simulink model "autoTakeoff"  (R2015a)
settings: Solver=ode45  StartTime=0.0  StopTime=inf  FixedStep=0.01  RelTol=1e-3
libraries: simulink x8, dspindex x8, dspnetwork x3, aerolibconvert2 x1, IMU_Library x1, GPS_Library x1, realtime_pacer_lib x1, etargetslib x1
settings Model: xpc_rtwmakecfg_data=_xpcnblib__xpcetherlib__xpcether8255xlib__xpcetherGbElib__xpciplib_  ParamWorkspaceSource=ReferencedWorkspace  CovSFcnEnable=off  Creator=abdkadma  LastModifiedBy=theth
settings OptimizationCC: InlineParams=on  InlineInvariantSignals=on  EnhancedBackFolding=on  ExpressionDepthLimit=2147483647  EfficientFloat2IntCast=on  SimCompilerOptimization=on
settings DebuggingCC: UnderspecifiedInitializationDetection=Classic  MergeDetectMultiDrivingBlocksExec=none  SolverPrmCheckMsg=warning  StateNameClashWarn=warning
settings RTWCC: RTWCompilerOptimization=on  CheckMdlBeforeBuild=Warning
settings GRTTargetCC: MatFileLogging=off  SupportNonFinite=off

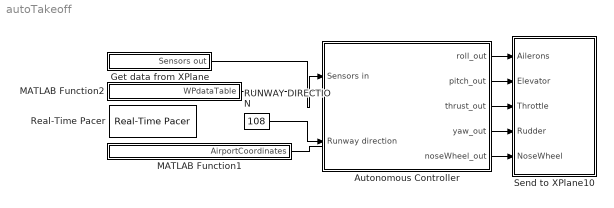
== system autoTakeoff ==
  "Autonomous Controller " : Subsystem
  Get data from XPlane : Subsystem  Description=|  TreatAsAtomicUnit=on  mask(Get Data from Xplane10){remoteURL='127.0.0.1', localPort=49005, sampletime=0.02}
      | Done by: Mohamed Abdelkader
      | Contact for updates: mohamedashraf123@gmail.com
      mask prompts: remoteURL "Remote IP address ('0.0.0.0' to accept all):(default='127.0.0.1')"; localPort "Local IP port: that Xplane10 sends to (default=49005)"; sampletime "Sampling time (seconds), how frequenlty to capture data from Xplane. Don't set to low as it might not be able to capture the smaples from Xplane. Default is 0.02 assuming the UDP rate in Xplane is set to 50 sample per second"
      mask help:
      | Get Data from X-Plane10
      | * make sure you configure the right port
      | and the right IP address
      mask TypeOptions remoteURL: UDP Receive1/remoteURL
      mask TypeOptions localPort: UDP Receive1/localPort
      mask TypeOptions sampletime: UDP Receive1/sampletime
  MATLAB Function1 : MATLAB Function  TreatAsAtomicUnit=on
  MATLAB Function2 : MATLAB Function  TreatAsAtomicUnit=on
  RUNWAY DIRECTION : Constant  Value=108
  Real-Time Pacer : realtime_pacer_lib/Real-Time Pacer  simTimePerRealTime=1
  Send to XPlane10 : Subsystem  Description=|  mask(Send Commands to X-Plane 10){remoteURL='127.0.0.1', remotePort=49000}
      | Done by: Mohamed Abdelkader
      | Contact for updates: mohamedashraf123@gmail.com
      mask prompts: remoteURL "Remote IP address (default='127.0.0.1'): X-Plane10 IP"; remotePort "Remote IP port:X-Plane10 port(default=49000)"
      mask help:
      | Sends Control Surfaces Commands to Xplane10
      | Throttle in [0,1]
      | Elevator, Ailerons, rudder, nosewheel in [-1,1]
      mask TypeOptions remoteURL: UDP Send/remoteURL
      mask TypeOptions remotePort: UDP Send/remotePort
  wires:
  "Autonomous Controller "/1(roll_out) -> Send to XPlane10/1(Ailerons)
  "Autonomous Controller "/2(pitch_out) -> Send to XPlane10/2(Elevator)
  "Autonomous Controller "/3(thrust_out) -> Send to XPlane10/3(Throttle)
  "Autonomous Controller "/4(yaw_out) -> Send to XPlane10/4(Rudder)
  "Autonomous Controller "/5(noseWheel_out) -> Send to XPlane10/5(NoseWheel)
  Get data from XPlane/1(Sensors out) -> "Autonomous Controller "/1(Sensors in)
  RUNWAY DIRECTION/1 -> "Autonomous Controller "/2(Runway direction)
  MATLAB Function1/1(AirportCoordinates) -> ?
  MATLAB Function2/1(WPdataTable) -> ?

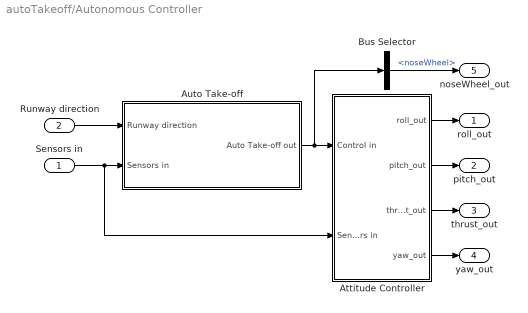
== system autoTakeoff/Autonomous Controller  ==
  Sensors in : Inport
  Runway direction : Inport  Port=2
  Attitude Controller : Subsystem
  Auto Take-off : Subsystem
  Bus Selector : BusSelector  OutputSignals=noseWheel
  roll_out : Outport
  pitch_out : Outport  Port=2
  thrust_out : Outport  Port=3
  yaw_out : Outport  Port=4
  noseWheel_out : Outport  Port=5
  wires:
  Attitude Controller/4(yaw_out) -> yaw_out/1
  Attitude Controller/1(roll_out) -> roll_out/1
  Attitude Controller/3(thrust_out) -> thrust_out/1
  Sensors in/1 -> Auto Take-off/2(Sensors in), Attitude Controller/2(Sensors in)
  Runway direction/1 -> Auto Take-off/1(Runway direction)
  Auto Take-off/1(Auto Take-off out) -> Attitude Controller/1(Control in), Bus Selector/1
  Attitude Controller/2(pitch_out) -> pitch_out/1
  Bus Selector/1 -> noseWheel_out/1  "<noseWheel>"

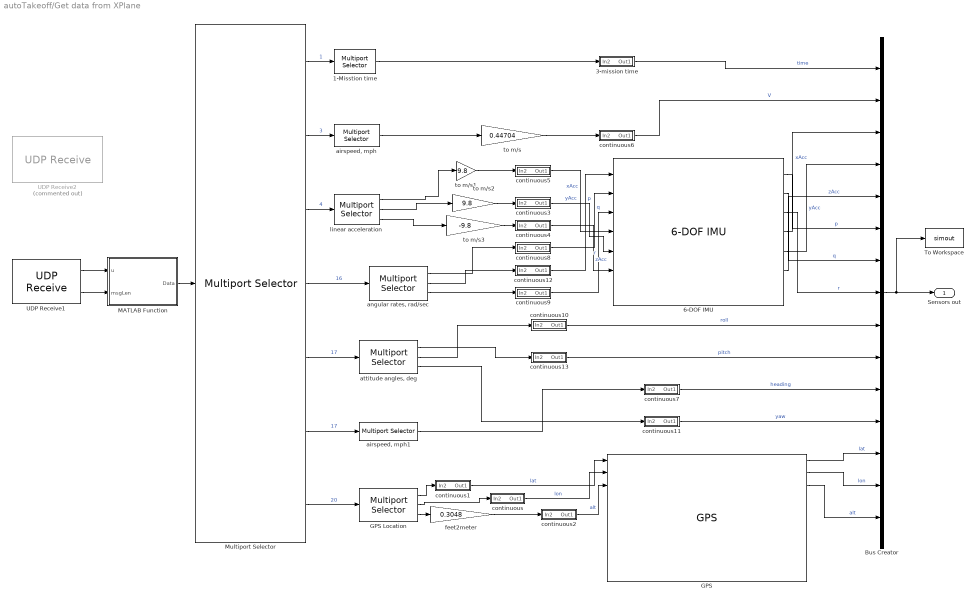
== system autoTakeoff/Get data from XPlane ==
  1-Misstion time : dspindex/Multiport Selector  rowsOrCols=Columns  idxCellArray={3}  idxErrMode=Clip Index
  3-mission time : Subsystem
  6-DOF IMU : IMU_Library/6-DOF IMU  lpf_filt_freq_hz_ix=20 Hz  gyro_scale_ix=+/- 500 deg/sec  accel_scale_ix=+/- 8g  SampleTime=0.02  lpf_filt_freq_hz=5 Hz  gyro_scale=+/- 250 deg/sec  accel_scale=+/- 2g
  Bus Creator : BusCreator  Inputs='time','V','xAcc','yAcc','zAcc','p','q','r','roll','pitch','heading','yaw','lat','lon','alt'
  GPS : GPS_Library/GPS
  GPS Location : dspindex/Multiport Selector  rowsOrCols=Columns  idxCellArray={1,2,3}  idxErrMode=Clip Index
  MATLAB Function : MATLAB Function  TreatAsAtomicUnit=on
  Multiport Selector : dspindex/Multiport Selector  rowsOrCols=Rows  idxCellArray={1,3,4,16,17,18,20}  idxErrMode=Clip Index
  To Workspace : ToWorkspace  VariableName=simout  SampleTime=-1
      settings: Save2DSignal=2-D array (concatenate along first dimension)
  UDP Receive1 : dspnetwork/UDP Receive  localURL='0.0.0.0'  localPort=localPort  remoteURL=remoteURL  remotePort=-1  recvBufferSize=8192  dims=365*20  signalDatatype=uint8  isVarSize=off  showBlockingTime=off  blockingTime=0  sampletime=sampletime
  UDP Receive2 : dspnetwork/UDP Receive  Commented=on  localURL='0.0.0.0'  localPort=localPort  remoteURL=remoteURL  remotePort=-1  recvBufferSize=8192  dims=365  signalDatatype=uint8  isVarSize=off  showBlockingTime=on  blockingTime=0.01  sampletime=0.01  blockPlatform=LINUX
  "airspeed, mph" : dspindex/Multiport Selector  rowsOrCols=Columns  idxCellArray={6}  idxErrMode=Clip Index
  "airspeed, mph1" : dspindex/Multiport Selector  rowsOrCols=Columns  idxCellArray={3}  idxErrMode=Clip Index
  "angular rates, rad/sec" : dspindex/Multiport Selector  rowsOrCols=Columns  idxCellArray={1,2,3}  idxErrMode=Clip Index
  "attitude angles, deg" : dspindex/Multiport Selector  rowsOrCols=Columns  idxCellArray={1,2,3}  idxErrMode=Clip Index
  continuous : Subsystem
  continuous1 : Subsystem
  continuous10 : Subsystem
  continuous11 : Subsystem
  continuous12 : Subsystem
  continuous13 : Subsystem
  continuous2 : Subsystem
  continuous3 : Subsystem
  continuous4 : Subsystem
  continuous5 : Subsystem
  continuous6 : Subsystem
  continuous7 : Subsystem
  continuous8 : Subsystem
  continuous9 : Subsystem
  feet2meter : Gain  Gain=0.3048
  linear acceleration : dspindex/Multiport Selector  rowsOrCols=Columns  idxCellArray={6,7,5}  idxErrMode=Clip Index
  to m/s : Gain  Gain=0.44704
  to m/s1 : Gain  Gain=9.8
  to m/s2 : Gain  Gain=9.8
  to m/s3 : Gain  Gain=-9.8
  Sensors out : Outport
  wires:
  "attitude angles, deg"/3 -> continuous11/1(In2)
  "angular rates, rad/sec"/3 -> continuous9/1(In2)
  MATLAB Function/1(Data) -> Multiport Selector/1
  linear acceleration/2 -> to m/s2/1
  to m/s2/1 -> continuous3/1(In2)
  to m/s1/1 -> continuous5/1(In2)
  "attitude angles, deg"/1 -> continuous13/1(In2)
  "attitude angles, deg"/2 -> continuous10/1(In2)
  to m/s/1 -> continuous6/1(In2)
  "airspeed, mph"/1 -> to m/s/1
  linear acceleration/1 -> to m/s1/1
  "angular rates, rad/sec"/1 -> continuous8/1(In2)
  linear acceleration/3 -> to m/s3/1
  "angular rates, rad/sec"/2 -> continuous12/1(In2)
  "airspeed, mph1"/1 -> continuous7/1(In2)
  to m/s3/1 -> continuous4/1(In2)
  feet2meter/1 -> continuous2/1(In2)
  UDP Receive1/1 -> MATLAB Function/1(u)
  UDP Receive1/2 -> MATLAB Function/2(msgLen)
  GPS Location/3 -> feet2meter/1
  GPS Location/1 -> continuous1/1(In2)
  continuous6/1(Out1) -> Bus Creator/2  "V"
  continuous7/1(Out1) -> Bus Creator/11  "heading"
  continuous10/1(Out1) -> Bus Creator/9  "roll"
  continuous11/1(Out1) -> Bus Creator/12  "yaw"
  continuous13/1(Out1) -> Bus Creator/10  "pitch"
  Bus Creator/1 -> To Workspace/1, Sensors out/1
  Multiport Selector/4 -> "angular rates, rad/sec"/1  "16"
  Multiport Selector/5 -> "attitude angles, deg"/1  "17"
  Multiport Selector/6 -> "airspeed, mph1"/1  "17"
  Multiport Selector/7 -> GPS Location/1  "20"
  1-Misstion time/1 -> 3-mission time/1(In2)
  3-mission time/1(Out1) -> Bus Creator/1  "time"
  Multiport Selector/1 -> 1-Misstion time/1  "1"
  Multiport Selector/2 -> "airspeed, mph"/1  "3"
  Multiport Selector/3 -> linear acceleration/1  "4"
  continuous5/1(Out1) -> 6-DOF IMU/4  "xAcc"
  6-DOF IMU/4 -> Bus Creator/3  "xAcc"
  continuous3/1(Out1) -> 6-DOF IMU/5  "yAcc"
  6-DOF IMU/5 -> Bus Creator/4  "yAcc"
  continuous4/1(Out1) -> 6-DOF IMU/6  "zAcc"
  6-DOF IMU/6 -> Bus Creator/5  "zAcc"
  continuous12/1(Out1) -> 6-DOF IMU/1  "p"
  continuous8/1(Out1) -> 6-DOF IMU/2  "q"
  continuous9/1(Out1) -> 6-DOF IMU/3  "r"
  6-DOF IMU/1 -> Bus Creator/6  "p"
  6-DOF IMU/2 -> Bus Creator/7  "q"
  6-DOF IMU/3 -> Bus Creator/8  "r"
  continuous1/1(Out1) -> GPS/1  "lat"
  GPS/1 -> Bus Creator/13  "lat"
  continuous/1(Out1) -> GPS/2  "lon"
  GPS/2 -> Bus Creator/14  "lon"
  continuous2/1(Out1) -> GPS/3  "alt"
  GPS/3 -> Bus Creator/15  "alt"
  GPS Location/2 -> continuous/1(In2)

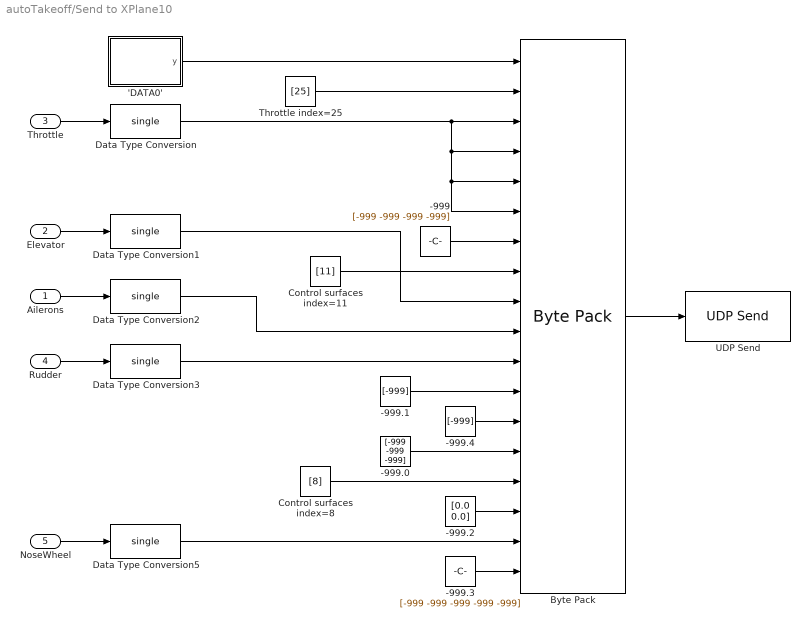
== system autoTakeoff/Send to XPlane10 ==
  Ailerons : Inport
  Elevator : Inport  Port=2
  Throttle : Inport  Port=3
  Rudder : Inport  Port=4
  NoseWheel : Inport  Port=5
  'DATA0' : MATLAB Function  TreatAsAtomicUnit=on
  -999 : Constant  Value=[-999 -999 -999 -999]  OutDataTypeStr=int32  SampleTime=-1
  -999.0 : Constant  Value=[-999 -999 -999]  OutDataTypeStr=int32  SampleTime=-1
  -999.1 : Constant  Value=[-999]  OutDataTypeStr=int32  SampleTime=-1
  -999.2 : Constant  Value=[0.0 0.0]  OutDataTypeStr=single  SampleTime=-1
  -999.3 : Constant  Value=[-999 -999 -999 -999 -999]  OutDataTypeStr=int32  SampleTime=-1
  -999.4 : Constant  Value=[-999]  OutDataTypeStr=single  SampleTime=-1
  Byte Pack : etargetslib/Byte Pack  datatypes={'uint8','uint32','single','single','single','single','int32','uint32','single','single','single','int32','single','int32','uint32','single','single','int32'}  byteAlign=1
  Control surfaces index=11 : Constant  Value=[11]  OutDataTypeStr=uint32  SampleTime=-1
  Control surfaces index=8 : Constant  Value=[8]  OutDataTypeStr=uint32  SampleTime=-1
  Data Type Conversion : DataTypeConversion  OutMin=[0]  OutMax=[1.0]  OutDataTypeStr=single
  Data Type Conversion{1..3,5} (4 alike) : DataTypeConversion  OutMin=[-1.0]  OutMax=[1.0]  OutDataTypeStr=single
  Throttle index=25 : Constant  Value=[25]  OutDataTypeStr=uint32  SampleTime=-1
  UDP Send : dspnetwork/UDP Send  remoteURL=remoteURL  remotePort=remotePort  localURL='0.0.0.0'  localPortSource=Automatically determine  localPort=-1  sampletime=-1  separateLengthPort=0
  wires:
  Ailerons/1 -> Data Type Conversion2/1
  Control surfaces index=11/1 -> Byte Pack/8
  Throttle/1 -> Data Type Conversion/1
  Data Type Conversion1/1 -> Byte Pack/9
  'DATA0'/1(y) -> Byte Pack/1
  Throttle index=25/1 -> Byte Pack/2
  Byte Pack/1 -> UDP Send/1
  -999/1 -> Byte Pack/7
  Data Type Conversion2/1 -> Byte Pack/10
  Data Type Conversion3/1 -> Byte Pack/11
  Rudder/1 -> Data Type Conversion3/1
  -999.0/1 -> Byte Pack/14
  Elevator/1 -> Data Type Conversion1/1
  Data Type Conversion/1 -> Byte Pack/3, Byte Pack/4, Byte Pack/6, Byte Pack/5
  -999.1/1 -> Byte Pack/12
  Control surfaces index=8/1 -> Byte Pack/15
  -999.2/1 -> Byte Pack/16
  Data Type Conversion5/1 -> Byte Pack/17
  NoseWheel/1 -> Data Type Conversion5/1
  -999.3/1 -> Byte Pack/18
  -999.4/1 -> Byte Pack/13

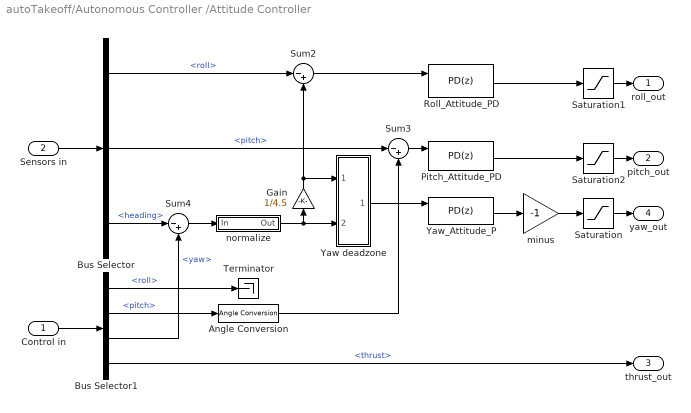
== system autoTakeoff/Autonomous Controller /Attitude Controller ==
  Control in : Inport
  Sensors in : Inport  Port=2
  Angle Conversion : aerolibconvert2/Angle Conversion  IU=rad  OU=deg
  Bus Selector : BusSelector  OutputSignals=roll,pitch,heading
  Bus Selector1 : BusSelector  OutputSignals=roll,pitch,yaw,thrust
  Gain : Gain  Gain=1/4.5
  Pitch_Attitude_PD : simulink/Continuous/PID Controller  Controller=PD  TimeDomain=Discrete-time  SampleTime=0.02  IntegratorMethod=Forward Euler  FilterMethod=Forward Euler  Form=Parallel  UseFilter=off  ControllerParametersSource=internal  P=1*pi/180  I=0  D=0.04*pi/180  N=20  InitialConditionSource=internal  InitialConditionForIntegrator=0  InitialConditionForFilter=0  ExternalReset=either  LimitOutput=on  UpperSaturationLimit=1  LowerSaturationLimit=-1  LinearizeAsGain=on  AntiWindupMode=none  Kb=1  TrackingMode=off  Kt=1  PParamMin=[]  PParamMax=[]  IParamMin=[]  IParamMax=[]  DParamMin=[]  DParamMax=[]  NParamMin=[]  NParamMax=[]  KbParamMin=[]  KbParamMax=[]  KtParamMin=[]  KtParamMax=[]  POutMin=[]  POutMax=[]  IOutMin=[]  IOutMax=[]  DOutMin=[]  DOutMax=[]  NOutMin=[]  NOutMax=[]  KbOutMin=[]  KbOutMax=[]  KtOutMin=[]  KtOutMax=[]  IntegratorOutMin=[]  IntegratorOutMax=[]  FilterOutMin=[]  FilterOutMax=[]  SumOutMin=[]  SumOutMax=[]  SumI1OutMin=[]  SumI1OutMax=[]  SumI2OutMin=[]  SumI2OutMax=[]  SumI3OutMin=[]  SumI3OutMax=[]  SumDOutMin=[]  SumDOutMax=[]  SaturationOutMin=[]  SaturationOutMax=[]  IntegratorContinuousStateAttributes=''  IntegratorStateMustResolveToSignalObject=off  IntegratorRTWStateStorageClass=Auto  FilterContinuousStateAttributes=''  FilterStateMustResolveToSignalObject=off  FilterRTWStateStorageClass=Auto  DifferentiatorICPrevScaledInput=0  DifferentiatorOutMin=[]  DifferentiatorOutMax=[]
  Roll_Attitude_PD : simulink/Continuous/PID Controller  Controller=PD  TimeDomain=Discrete-time  SampleTime=0.02  IntegratorMethod=Forward Euler  FilterMethod=Forward Euler  Form=Parallel  UseFilter=off  ControllerParametersSource=internal  P=pi/180/4  I=0  D=0.0008*pi/180/4  N=20  InitialConditionSource=internal  InitialConditionForIntegrator=0  InitialConditionForFilter=0  ExternalReset=either  LimitOutput=on  UpperSaturationLimit=1  LowerSaturationLimit=-1  LinearizeAsGain=on  AntiWindupMode=none  Kb=1  TrackingMode=off  Kt=1  PParamMin=[]  PParamMax=[]  IParamMin=[]  IParamMax=[]  DParamMin=[]  DParamMax=[]  NParamMin=[]  NParamMax=[]  KbParamMin=[]  KbParamMax=[]  KtParamMin=[]  KtParamMax=[]  POutMin=[]  POutMax=[]  IOutMin=[]  IOutMax=[]  DOutMin=[]  DOutMax=[]  NOutMin=[]  NOutMax=[]  KbOutMin=[]  KbOutMax=[]  KtOutMin=[]  KtOutMax=[]  IntegratorOutMin=[]  IntegratorOutMax=[]  FilterOutMin=[]  FilterOutMax=[]  SumOutMin=[]  SumOutMax=[]  SumI1OutMin=[]  SumI1OutMax=[]  SumI2OutMin=[]  SumI2OutMax=[]  SumI3OutMin=[]  SumI3OutMax=[]  SumDOutMin=[]  SumDOutMax=[]  SaturationOutMin=[]  SaturationOutMax=[]  IntegratorContinuousStateAttributes=''  IntegratorStateMustResolveToSignalObject=off  IntegratorRTWStateStorageClass=Auto  FilterContinuousStateAttributes=''  FilterStateMustResolveToSignalObject=off  FilterRTWStateStorageClass=Auto  DifferentiatorICPrevScaledInput=0  DifferentiatorOutMin=[]  DifferentiatorOutMax=[]
  Saturation : Saturate  UpperLimit=1  LowerLimit=-1
  Saturation1 : Saturate  UpperLimit=0.05  LowerLimit=-0.05
  Saturation2 : Saturate  UpperLimit=1  LowerLimit=-1
  Sum2 : Sum  Inputs=|-+
  Sum3 : Sum  Inputs=|-+
  Sum4 : Sum  Inputs=|-+
  Terminator : Terminator
  Yaw deadzone : Subsystem
  Yaw_Attitude_P : simulink/Continuous/PID Controller  Controller=PD  TimeDomain=Discrete-time  SampleTime=0.02  IntegratorMethod=Forward Euler  FilterMethod=Forward Euler  Form=Parallel  UseFilter=off  ControllerParametersSource=internal  P=6*pi/180  I=0  D=6*0.000034  N=100  InitialConditionSource=internal  InitialConditionForIntegrator=0  InitialConditionForFilter=0  ExternalReset=either  LimitOutput=on  UpperSaturationLimit=1  LowerSaturationLimit=-1  LinearizeAsGain=on  AntiWindupMode=none  Kb=1  TrackingMode=off  Kt=1  PParamMin=[]  PParamMax=[]  IParamMin=[]  IParamMax=[]  DParamMin=[]  DParamMax=[]  NParamMin=[]  NParamMax=[]  KbParamMin=[]  KbParamMax=[]  KtParamMin=[]  KtParamMax=[]  POutMin=[]  POutMax=[]  IOutMin=[]  IOutMax=[]  DOutMin=[]  DOutMax=[]  NOutMin=[]  NOutMax=[]  KbOutMin=[]  KbOutMax=[]  KtOutMin=[]  KtOutMax=[]  IntegratorOutMin=[]  IntegratorOutMax=[]  FilterOutMin=[]  FilterOutMax=[]  SumOutMin=[]  SumOutMax=[]  SumI1OutMin=[]  SumI1OutMax=[]  SumI2OutMin=[]  SumI2OutMax=[]  SumI3OutMin=[]  SumI3OutMax=[]  SumDOutMin=[]  SumDOutMax=[]  SaturationOutMin=[]  SaturationOutMax=[]  IntegratorContinuousStateAttributes=''  IntegratorStateMustResolveToSignalObject=off  IntegratorRTWStateStorageClass=Auto  FilterContinuousStateAttributes=''  FilterStateMustResolveToSignalObject=off  FilterRTWStateStorageClass=Auto  DifferentiatorICPrevScaledInput=0  DifferentiatorOutMin=[]  DifferentiatorOutMax=[]
  minus : Gain  Gain=-1
  normalize : Subsystem
  roll_out : Outport
  pitch_out : Outport  Port=2
  thrust_out : Outport  Port=3
  yaw_out : Outport  Port=4
  wires:
  Sum2/1 -> Roll_Attitude_PD/1
  Sum3/1 -> Pitch_Attitude_PD/1
  Bus Selector/1 -> Sum2/1  "<roll>"
  Bus Selector/2 -> Sum3/1  "<pitch>"
  minus/1 -> Saturation/1
  Bus Selector/3 -> Sum4/1  "<heading>"
  Sum4/1 -> normalize/1(In)
  Sensors in/1 -> Bus Selector/1
  Control in/1 -> Bus Selector1/1
  Bus Selector1/2 -> Angle Conversion/1  "<pitch>"
  Bus Selector1/4 -> thrust_out/1  "<thrust>"
  Bus Selector1/3 -> Sum4/2  "<yaw>"
  Saturation1/1 -> roll_out/1
  Saturation2/1 -> pitch_out/1
  Yaw_Attitude_P/1 -> minus/1
  Pitch_Attitude_PD/1 -> Saturation2/1
  Roll_Attitude_PD/1 -> Saturation1/1
  Saturation/1 -> yaw_out/1
  Gain/1 -> Sum2/2, Yaw deadzone/1(Roll)
  Angle Conversion/1 -> Sum3/2
  normalize/1(Out) -> Gain/1, Yaw deadzone/2(in)
  Yaw deadzone/1(out) -> Yaw_Attitude_P/1
  Bus Selector1/1 -> Terminator/1  "<roll>"

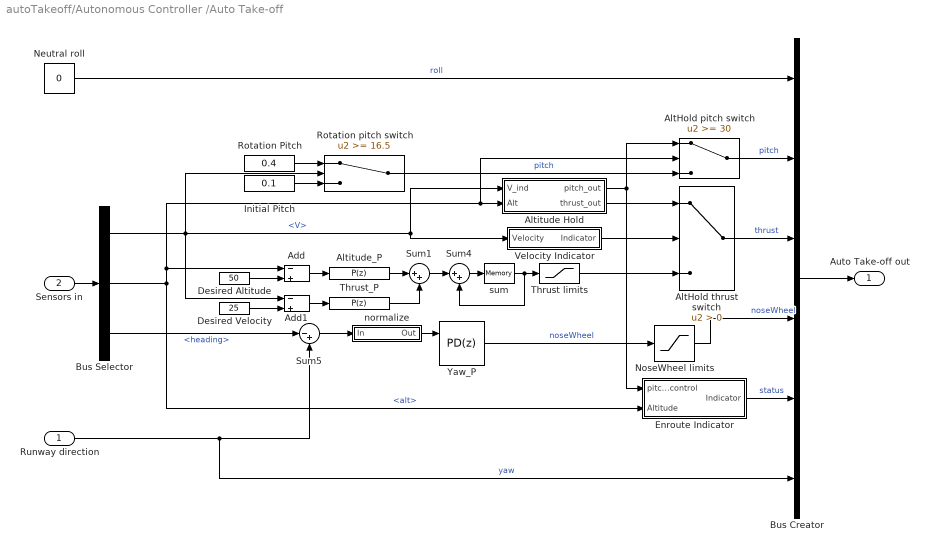
== system autoTakeoff/Autonomous Controller /Auto Take-off ==
  Runway direction : Inport
  Sensors in : Inport  Port=2
  Add : Sum  Inputs=-+
  Add1 : Sum  Inputs=-+
  AltHold pitch switch : Switch  Threshold=30
  AltHold thrust switch : Switch  Criteria=u2 > Threshold
  Altitude Hold : Subsystem
  Altitude_P : simulink/Continuous/PID Controller  Controller=P  TimeDomain=Discrete-time  SampleTime=-1  IntegratorMethod=Forward Euler  FilterMethod=Forward Euler  Form=Parallel  UseFilter=on  ControllerParametersSource=internal  P=0.1  I=0  D=0.01  N=20  InitialConditionSource=internal  InitialConditionForIntegrator=0  InitialConditionForFilter=0  ExternalReset=either  LimitOutput=on  UpperSaturationLimit=1  LowerSaturationLimit=-1  LinearizeAsGain=on  AntiWindupMode=none  Kb=1  TrackingMode=off  Kt=1  PParamMin=[]  PParamMax=[]  IParamMin=[]  IParamMax=[]  DParamMin=[]  DParamMax=[]  NParamMin=[]  NParamMax=[]  KbParamMin=[]  KbParamMax=[]  KtParamMin=[]  KtParamMax=[]  POutMin=[]  POutMax=[]  IOutMin=[]  IOutMax=[]  DOutMin=[]  DOutMax=[]  NOutMin=[]  NOutMax=[]  KbOutMin=[]  KbOutMax=[]  KtOutMin=[]  KtOutMax=[]  IntegratorOutMin=[]  IntegratorOutMax=[]  FilterOutMin=[]  FilterOutMax=[]  SumOutMin=[]  SumOutMax=[]  SumI1OutMin=[]  SumI1OutMax=[]  SumI2OutMin=[]  SumI2OutMax=[]  SumI3OutMin=[]  SumI3OutMax=[]  SumDOutMin=[]  SumDOutMax=[]  SaturationOutMin=[]  SaturationOutMax=[]  IntegratorContinuousStateAttributes=''  IntegratorStateMustResolveToSignalObject=off  IntegratorRTWStateStorageClass=Auto  FilterContinuousStateAttributes=''  FilterStateMustResolveToSignalObject=off  FilterRTWStateStorageClass=Auto  DifferentiatorICPrevScaledInput=0  DifferentiatorOutMin=[]  DifferentiatorOutMax=[]
  Bus Creator : BusCreator  Inputs='roll','pitch','thrust','noseWheel','status','yaw'
  Bus Selector : BusSelector  OutputSignals=V,alt,heading
  Desired Altitude : Constant  Value=50  OutDataTypeStr=single
  Desired Velocity : Constant  Value=25  OutDataTypeStr=single
  Enroute Indicator : Subsystem
  Initial Pitch : Constant  Value=0.1  OutDataTypeStr=single
  Neutral roll : Constant  Value=0  OutDataTypeStr=single
  NoseWheel limits : Saturate
  Rotation Pitch : Constant  Value=0.4  OutDataTypeStr=single
  Rotation pitch switch : Switch  Threshold=16.5
  Sum1 : Sum  Inputs=|++
  Sum4 : Sum  Inputs=|++
  Sum5 : Sum  Inputs=|-+
  Thrust limits : Saturate  UpperLimit=1  LowerLimit=0
  Thrust_P : simulink/Continuous/PID Controller  Controller=P  TimeDomain=Discrete-time  SampleTime=-1  IntegratorMethod=Forward Euler  FilterMethod=Forward Euler  Form=Parallel  UseFilter=on  ControllerParametersSource=internal  P=0.1  I=0  D=0.01  N=20  InitialConditionSource=internal  InitialConditionForIntegrator=0  InitialConditionForFilter=0  ExternalReset=either  LimitOutput=on  UpperSaturationLimit=1  LowerSaturationLimit=-1  LinearizeAsGain=on  AntiWindupMode=none  Kb=1  TrackingMode=off  Kt=1  PParamMin=[]  PParamMax=[]  IParamMin=[]  IParamMax=[]  DParamMin=[]  DParamMax=[]  NParamMin=[]  NParamMax=[]  KbParamMin=[]  KbParamMax=[]  KtParamMin=[]  KtParamMax=[]  POutMin=[]  POutMax=[]  IOutMin=[]  IOutMax=[]  DOutMin=[]  DOutMax=[]  NOutMin=[]  NOutMax=[]  KbOutMin=[]  KbOutMax=[]  KtOutMin=[]  KtOutMax=[]  IntegratorOutMin=[]  IntegratorOutMax=[]  FilterOutMin=[]  FilterOutMax=[]  SumOutMin=[]  SumOutMax=[]  SumI1OutMin=[]  SumI1OutMax=[]  SumI2OutMin=[]  SumI2OutMax=[]  SumI3OutMin=[]  SumI3OutMax=[]  SumDOutMin=[]  SumDOutMax=[]  SaturationOutMin=[]  SaturationOutMax=[]  IntegratorContinuousStateAttributes=''  IntegratorStateMustResolveToSignalObject=off  IntegratorRTWStateStorageClass=Auto  FilterContinuousStateAttributes=''  FilterStateMustResolveToSignalObject=off  FilterRTWStateStorageClass=Auto  DifferentiatorICPrevScaledInput=0  DifferentiatorOutMin=[]  DifferentiatorOutMax=[]
  Velocity Indicator : Subsystem
  Yaw_P : simulink/Continuous/PID Controller  Controller=PD  TimeDomain=Discrete-time  SampleTime=0.02  IntegratorMethod=Forward Euler  FilterMethod=Forward Euler  Form=Parallel  UseFilter=off  ControllerParametersSource=internal  P=0.012  I=0  D=0.0024  N=100  InitialConditionSource=internal  InitialConditionForIntegrator=0  InitialConditionForFilter=0  ExternalReset=either  LimitOutput=on  UpperSaturationLimit=1  LowerSaturationLimit=-1  LinearizeAsGain=on  AntiWindupMode=none  Kb=1  TrackingMode=off  Kt=1  PParamMin=[]  PParamMax=[]  IParamMin=[]  IParamMax=[]  DParamMin=[]  DParamMax=[]  NParamMin=[]  NParamMax=[]  KbParamMin=[]  KbParamMax=[]  KtParamMin=[]  KtParamMax=[]  POutMin=[]  POutMax=[]  IOutMin=[]  IOutMax=[]  DOutMin=[]  DOutMax=[]  NOutMin=[]  NOutMax=[]  KbOutMin=[]  KbOutMax=[]  KtOutMin=[]  KtOutMax=[]  IntegratorOutMin=[]  IntegratorOutMax=[]  FilterOutMin=[]  FilterOutMax=[]  SumOutMin=[]  SumOutMax=[]  SumI1OutMin=[]  SumI1OutMax=[]  SumI2OutMin=[]  SumI2OutMax=[]  SumI3OutMin=[]  SumI3OutMax=[]  SumDOutMin=[]  SumDOutMax=[]  SaturationOutMin=[]  SaturationOutMax=[]  IntegratorContinuousStateAttributes=''  IntegratorStateMustResolveToSignalObject=off  IntegratorRTWStateStorageClass=Auto  FilterContinuousStateAttributes=''  FilterStateMustResolveToSignalObject=off  FilterRTWStateStorageClass=Auto  DifferentiatorICPrevScaledInput=0  DifferentiatorOutMin=[]  DifferentiatorOutMax=[]
  normalize : Subsystem
  sum : Memory
  Auto Take-off out : Outport
  wires:
  Rotation Pitch/1 -> Rotation pitch switch/1
  Initial Pitch/1 -> Rotation pitch switch/3
  Neutral roll/1 -> Bus Creator/1  "roll"
  Add1/1 -> Thrust_P/1
  Desired Velocity/1 -> Add1/2
  Altitude_P/1 -> Sum1/1
  Add/1 -> Altitude_P/1
  Desired Altitude/1 -> Add/2
  sum/1 -> Sum4/2, Thrust limits/1
  Sum4/1 -> sum/1
  Bus Selector/3 -> Sum5/1  "<heading>"
  Runway direction/1 -> Sum5/2, Bus Creator/6  "yaw"
  Bus Selector/2 -> AltHold pitch switch/2, Altitude Hold/2(Alt), Add/1, Enroute Indicator/2(Altitude)  "<alt>"
  Bus Selector/1 -> Rotation pitch switch/2, Altitude Hold/1(V_ind), Velocity Indicator/1(Velocity), Add1/1  "<V>"
  Sum5/1 -> normalize/1(In)
  normalize/1(Out) -> Yaw_P/1
  Enroute Indicator/1(Indicator) -> Bus Creator/5  "status"
  Bus Creator/1 -> Auto Take-off out/1
  Sensors in/1 -> Bus Selector/1
  AltHold pitch switch/1 -> Bus Creator/2  "pitch"
  Rotation pitch switch/1 -> AltHold pitch switch/3  "pitch"
  Sum1/1 -> Sum4/1
  Thrust_P/1 -> Sum1/2
  AltHold thrust switch/1 -> Bus Creator/3  "thrust"
  Altitude Hold/2(thrust_out) -> AltHold thrust switch/1
  Altitude Hold/1(pitch_out) -> Enroute Indicator/1(pitch control), AltHold pitch switch/1
  Velocity Indicator/1(Indicator) -> AltHold thrust switch/2
  Yaw_P/1 -> NoseWheel limits/1  "noseWheel"
  Thrust limits/1 -> AltHold thrust switch/3
  NoseWheel limits/1 -> Bus Creator/4  "noseWheel"

== system autoTakeoff/Get data from XPlane/3-mission time ==
  In2 : Inport
  Memory2 : Memory
  Switch2 : Switch  Criteria=u2 ~= 0
  Out1 : Outport
  wires:
  Memory2/1 -> Switch2/3, Out1/1
  Switch2/1 -> Memory2/1
  In2/1 -> Switch2/1, Switch2/2

== system autoTakeoff/Get data from XPlane/continuous ==
  In2 : Inport
  Memory2 : Memory
  Switch2 : Switch  Criteria=u2 ~= 0
  Out1 : Outport
  wires:
  Memory2/1 -> Switch2/3, Out1/1
  Switch2/1 -> Memory2/1
  In2/1 -> Switch2/1, Switch2/2

== system autoTakeoff/Get data from XPlane/continuous1 ==
  In2 : Inport
  Memory2 : Memory
  Switch2 : Switch  Criteria=u2 ~= 0
  Out1 : Outport
  wires:
  Memory2/1 -> Switch2/3, Out1/1
  Switch2/1 -> Memory2/1
  In2/1 -> Switch2/1, Switch2/2

== system autoTakeoff/Get data from XPlane/continuous10 ==
  In2 : Inport
  Memory2 : Memory
  Switch2 : Switch  Criteria=u2 ~= 0
  Out1 : Outport
  wires:
  Memory2/1 -> Switch2/3, Out1/1
  Switch2/1 -> Memory2/1
  In2/1 -> Switch2/1, Switch2/2

== system autoTakeoff/Get data from XPlane/continuous11 ==
  In2 : Inport
  Memory2 : Memory
  Switch2 : Switch  Criteria=u2 ~= 0
  Out1 : Outport
  wires:
  Memory2/1 -> Switch2/3, Out1/1
  Switch2/1 -> Memory2/1
  In2/1 -> Switch2/1, Switch2/2

== system autoTakeoff/Get data from XPlane/continuous12 ==
  In2 : Inport
  Memory2 : Memory
  Switch2 : Switch  Criteria=u2 ~= 0
  Out1 : Outport
  wires:
  Memory2/1 -> Switch2/3, Out1/1
  Switch2/1 -> Memory2/1
  In2/1 -> Switch2/1, Switch2/2

== system autoTakeoff/Get data from XPlane/continuous13 ==
  In2 : Inport
  Memory2 : Memory
  Switch2 : Switch  Criteria=u2 ~= 0
  Out1 : Outport
  wires:
  Memory2/1 -> Switch2/3, Out1/1
  Switch2/1 -> Memory2/1
  In2/1 -> Switch2/1, Switch2/2

== system autoTakeoff/Get data from XPlane/continuous2 ==
  In2 : Inport
  Memory2 : Memory
  Switch2 : Switch  Criteria=u2 ~= 0
  Out1 : Outport
  wires:
  Memory2/1 -> Switch2/3, Out1/1
  Switch2/1 -> Memory2/1
  In2/1 -> Switch2/1, Switch2/2

== system autoTakeoff/Get data from XPlane/continuous3 ==
  In2 : Inport
  Memory2 : Memory
  Switch2 : Switch  Criteria=u2 ~= 0
  Out1 : Outport
  wires:
  Memory2/1 -> Switch2/3, Out1/1
  Switch2/1 -> Memory2/1
  In2/1 -> Switch2/1, Switch2/2

== system autoTakeoff/Get data from XPlane/continuous4 ==
  In2 : Inport
  Memory2 : Memory
  Switch2 : Switch  Criteria=u2 ~= 0
  Out1 : Outport
  wires:
  Memory2/1 -> Switch2/3, Out1/1
  Switch2/1 -> Memory2/1
  In2/1 -> Switch2/1, Switch2/2

== system autoTakeoff/Get data from XPlane/continuous5 ==
  In2 : Inport
  Memory2 : Memory
  Switch2 : Switch  Criteria=u2 ~= 0
  Out1 : Outport
  wires:
  Memory2/1 -> Switch2/3, Out1/1
  Switch2/1 -> Memory2/1
  In2/1 -> Switch2/1, Switch2/2

== system autoTakeoff/Get data from XPlane/continuous6 ==
  In2 : Inport
  Memory2 : Memory
  Switch2 : Switch  Criteria=u2 ~= 0
  Out1 : Outport
  wires:
  Memory2/1 -> Switch2/3, Out1/1
  Switch2/1 -> Memory2/1
  In2/1 -> Switch2/1, Switch2/2

== system autoTakeoff/Get data from XPlane/continuous7 ==
  In2 : Inport
  Memory2 : Memory
  Switch2 : Switch  Criteria=u2 ~= 0
  Out1 : Outport
  wires:
  Memory2/1 -> Switch2/3, Out1/1
  Switch2/1 -> Memory2/1
  In2/1 -> Switch2/1, Switch2/2

== system autoTakeoff/Get data from XPlane/continuous8 ==
  In2 : Inport
  Memory2 : Memory
  Switch2 : Switch  Criteria=u2 ~= 0
  Out1 : Outport
  wires:
  Memory2/1 -> Switch2/3, Out1/1
  Switch2/1 -> Memory2/1
  In2/1 -> Switch2/1, Switch2/2

== system autoTakeoff/Get data from XPlane/continuous9 ==
  In2 : Inport
  Memory2 : Memory
  Switch2 : Switch  Criteria=u2 ~= 0
  Out1 : Outport
  wires:
  Memory2/1 -> Switch2/3, Out1/1
  Switch2/1 -> Memory2/1
  In2/1 -> Switch2/1, Switch2/2

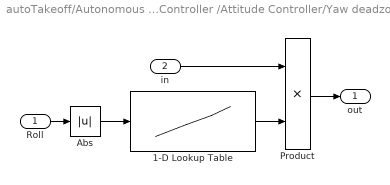
== system autoTakeoff/Autonomous Controller /Attitude Controller/Yaw deadzone ==
  Roll : Inport
  in : Inport  Port=2
  1-D Lookup Table : Lookup_n-D  NumberOfTableDimensions=1  BreakpointsForDimension1=[0,5,7,10,12.5,15,17,40]  BreakpointsForDimension2=[10,13,17,23,30,40,50]  Table=[1,0.30329,0.16957,0.07655,0.033915,0.010659,0,0]  InternalRulePriority=Speed  RndMeth=Simplest  InputSameDT=on
  Abs : Abs
  Product : Product
  out : Outport
  wires:
  Abs/1 -> 1-D Lookup Table/1
  Roll/1 -> Abs/1
  in/1 -> Product/1
  Product/1 -> out/1
  1-D Lookup Table/1 -> Product/2

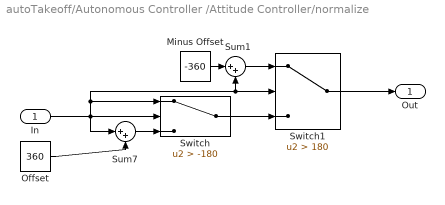
== system autoTakeoff/Autonomous Controller /Attitude Controller/normalize ==
  In : Inport
  Minus Offset : Constant  Value=-360
  Offset : Constant  Value=360
  Sum1 : Sum  Inputs=|++
  Sum7 : Sum  Inputs=|++
  Switch : Switch  Criteria=u2 > Threshold  Threshold=-180
  Switch1 : Switch  Criteria=u2 > Threshold  Threshold=180
  Out : Outport
  wires:
  Offset/1 -> Sum7/2
  Sum7/1 -> Switch/3
  In/1 -> Switch/2, Switch/1, Sum1/2, Switch1/2, Sum7/1
  Sum1/1 -> Switch1/1
  Minus Offset/1 -> Sum1/1
  Switch/1 -> Switch1/3
  Switch1/1 -> Out/1

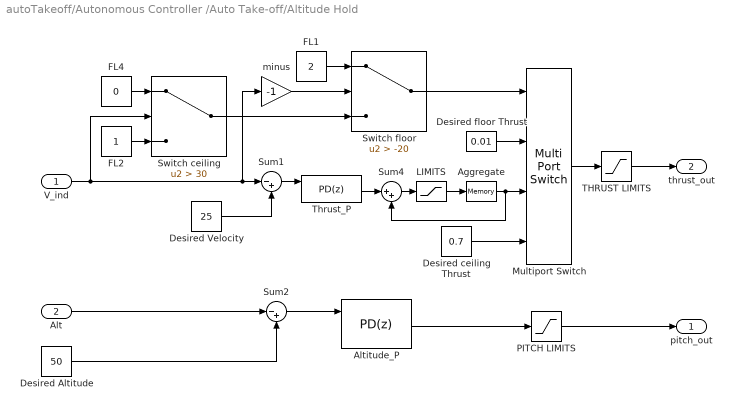
== system autoTakeoff/Autonomous Controller /Auto Take-off/Altitude Hold ==
  V_ind : Inport
  Alt : Inport  Port=2
  Aggregate : Memory
  Altitude_P : simulink/Continuous/PID Controller  Controller=PD  TimeDomain=Discrete-time  SampleTime=0.02  IntegratorMethod=Forward Euler  FilterMethod=Forward Euler  Form=Parallel  UseFilter=off  ControllerParametersSource=internal  P=0.12  I=0.0003  D=0.0024  N=20  InitialConditionSource=internal  InitialConditionForIntegrator=0  InitialConditionForFilter=0  ExternalReset=either  LimitOutput=on  UpperSaturationLimit=1  LowerSaturationLimit=-1  LinearizeAsGain=on  AntiWindupMode=none  Kb=1  TrackingMode=off  Kt=1  PParamMin=[]  PParamMax=[]  IParamMin=[]  IParamMax=[]  DParamMin=[]  DParamMax=[]  NParamMin=[]  NParamMax=[]  KbParamMin=[]  KbParamMax=[]  KtParamMin=[]  KtParamMax=[]  POutMin=[]  POutMax=[]  IOutMin=[]  IOutMax=[]  DOutMin=[]  DOutMax=[]  NOutMin=[]  NOutMax=[]  KbOutMin=[]  KbOutMax=[]  KtOutMin=[]  KtOutMax=[]  IntegratorOutMin=[]  IntegratorOutMax=[]  FilterOutMin=[]  FilterOutMax=[]  SumOutMin=[]  SumOutMax=[]  SumI1OutMin=[]  SumI1OutMax=[]  SumI2OutMin=[]  SumI2OutMax=[]  SumI3OutMin=[]  SumI3OutMax=[]  SumDOutMin=[]  SumDOutMax=[]  SaturationOutMin=[]  SaturationOutMax=[]  IntegratorContinuousStateAttributes=''  IntegratorStateMustResolveToSignalObject=off  IntegratorRTWStateStorageClass=Auto  FilterContinuousStateAttributes=''  FilterStateMustResolveToSignalObject=off  FilterRTWStateStorageClass=Auto  DifferentiatorICPrevScaledInput=0  DifferentiatorOutMin=[]  DifferentiatorOutMax=[]
  Desired Altitude : Constant  Value=50  OutDataTypeStr=single
  Desired Velocity : Constant  Value=25  OutDataTypeStr=single
  "Desired ceiling Thrust " : Constant  Value=0.7  OutDataTypeStr=single
  Desired floor Thrust : Constant  Value=0.01  OutDataTypeStr=single
  FL1 : Constant  Value=2  OutDataTypeStr=single
  FL2 : Constant  OutDataTypeStr=single
  FL4 : Constant  Value=0  OutDataTypeStr=single
  LIMITS : Saturate  UpperLimit=0.4  LowerLimit=0
  Multiport Switch : MultiPortSwitch  DataPortOrder=Zero-based contiguous
  PITCH LIMITS : Saturate  UpperLimit=0.2  LowerLimit=-0.2
  Sum1 : Sum  Inputs=|-+
  Sum2 : Sum  Inputs=|-+
  Sum4 : Sum  Inputs=|++
  Switch ceiling : Switch  Criteria=u2 > Threshold  Threshold=30
  Switch floor : Switch  Criteria=u2 > Threshold  Threshold=-20
  THRUST LIMITS : Saturate  UpperLimit=1  LowerLimit=0
  Thrust_P : simulink/Continuous/PID Controller  Controller=PD  TimeDomain=Discrete-time  SampleTime=0.02  IntegratorMethod=Forward Euler  FilterMethod=Forward Euler  Form=Parallel  UseFilter=off  ControllerParametersSource=internal  P=0.0005  I=0.0000000001  D=0.003  N=20  InitialConditionSource=internal  InitialConditionForIntegrator=0  InitialConditionForFilter=0  ExternalReset=either  LimitOutput=on  UpperSaturationLimit=1  LowerSaturationLimit=-1  LinearizeAsGain=on  AntiWindupMode=none  Kb=1  TrackingMode=off  Kt=1  PParamMin=[]  PParamMax=[]  IParamMin=[]  IParamMax=[]  DParamMin=[]  DParamMax=[]  NParamMin=[]  NParamMax=[]  KbParamMin=[]  KbParamMax=[]  KtParamMin=[]  KtParamMax=[]  POutMin=[]  POutMax=[]  IOutMin=[]  IOutMax=[]  DOutMin=[]  DOutMax=[]  NOutMin=[]  NOutMax=[]  KbOutMin=[]  KbOutMax=[]  KtOutMin=[]  KtOutMax=[]  IntegratorOutMin=[]  IntegratorOutMax=[]  FilterOutMin=[]  FilterOutMax=[]  SumOutMin=[]  SumOutMax=[]  SumI1OutMin=[]  SumI1OutMax=[]  SumI2OutMin=[]  SumI2OutMax=[]  SumI3OutMin=[]  SumI3OutMax=[]  SumDOutMin=[]  SumDOutMax=[]  SaturationOutMin=[]  SaturationOutMax=[]  IntegratorContinuousStateAttributes=''  IntegratorStateMustResolveToSignalObject=off  IntegratorRTWStateStorageClass=Auto  FilterContinuousStateAttributes=''  FilterStateMustResolveToSignalObject=off  FilterRTWStateStorageClass=Auto  DifferentiatorICPrevScaledInput=0  DifferentiatorOutMin=[]  DifferentiatorOutMax=[]
  minus : Gain  Gain=-1
  pitch_out : Outport
  thrust_out : Outport  Port=2
  wires:
  PITCH LIMITS/1 -> pitch_out/1
  Sum2/1 -> Altitude_P/1
  Desired Altitude/1 -> Sum2/2
  Altitude_P/1 -> PITCH LIMITS/1
  Sum1/1 -> Thrust_P/1
  Desired Velocity/1 -> Sum1/2
  Sum4/1 -> LIMITS/1
  Thrust_P/1 -> Sum4/1
  Alt/1 -> Sum2/1
  Switch ceiling/1 -> Switch floor/3
  V_ind/1 -> Switch ceiling/2, minus/1, Sum1/1
  minus/1 -> Switch floor/2
  Switch floor/1 -> Multiport Switch/1
  FL1/1 -> Switch floor/1
  Desired floor Thrust/1 -> Multiport Switch/2
  Multiport Switch/1 -> THRUST LIMITS/1
  FL4/1 -> Switch ceiling/1
  FL2/1 -> Switch ceiling/3
  "Desired ceiling Thrust "/1 -> Multiport Switch/4
  THRUST LIMITS/1 -> thrust_out/1
  LIMITS/1 -> Aggregate/1
  Aggregate/1 -> Multiport Switch/3, Sum4/2

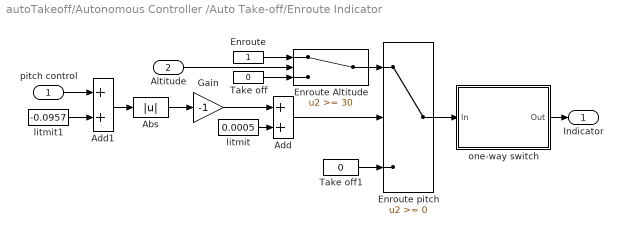
== system autoTakeoff/Autonomous Controller /Auto Take-off/Enroute Indicator ==
  pitch control : Inport
  Altitude : Inport  Port=2
  Abs : Abs
  Add : Sum
  Add1 : Sum
  Enroute : Constant  OutDataTypeStr=single
  Enroute Altitude : Switch  Threshold=30
  Enroute pitch : Switch
  Gain : Gain  Gain=-1
  Take off : Constant  Value=0  OutDataTypeStr=single
  Take off1 : Constant  Value=0  OutDataTypeStr=single
  litmit : Constant  Value=0.0005
  litmit1 : Constant  Value=-0.0957
  "one-way switch " : Subsystem
  Indicator : Outport
  wires:
  Enroute/1 -> Enroute Altitude/1
  Take off/1 -> Enroute Altitude/3
  Altitude/1 -> Enroute Altitude/2
  "one-way switch "/1(Out) -> Indicator/1
  Abs/1 -> Gain/1
  litmit/1 -> Add/2
  Add/1 -> Enroute pitch/2
  Gain/1 -> Add/1
  Enroute Altitude/1 -> Enroute pitch/1
  Take off1/1 -> Enroute pitch/3
  Enroute pitch/1 -> "one-way switch "/1(In)
  pitch control/1 -> Add1/1
  litmit1/1 -> Add1/2
  Add1/1 -> Abs/1

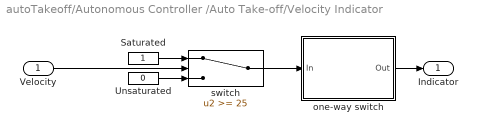
== system autoTakeoff/Autonomous Controller /Auto Take-off/Velocity Indicator ==
  Velocity : Inport
  Saturated : Constant  OutDataTypeStr=single
  Unsaturated : Constant  Value=0  OutDataTypeStr=single
  "one-way switch " : Subsystem
  switch : Switch  Threshold=25
  Indicator : Outport
  wires:
  Saturated/1 -> switch/1
  Unsaturated/1 -> switch/3
  Velocity/1 -> switch/2
  "one-way switch "/1(Out) -> Indicator/1
  switch/1 -> "one-way switch "/1(In)

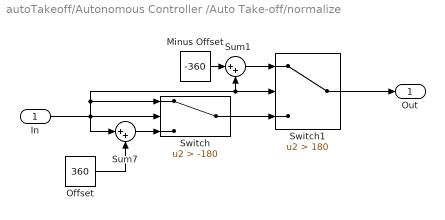
== system autoTakeoff/Autonomous Controller /Auto Take-off/normalize ==
  In : Inport
  Minus Offset : Constant  Value=-360
  Offset : Constant  Value=360
  Sum1 : Sum  Inputs=|++
  Sum7 : Sum  Inputs=|++
  Switch : Switch  Criteria=u2 > Threshold  Threshold=-180
  Switch1 : Switch  Criteria=u2 > Threshold  Threshold=180
  Out : Outport
  wires:
  Offset/1 -> Sum7/2
  Sum7/1 -> Switch/3
  In/1 -> Switch/2, Switch/1, Sum1/2, Switch1/2, Sum7/1
  Sum1/1 -> Switch1/1
  Minus Offset/1 -> Sum1/1
  Switch/1 -> Switch1/3
  Switch1/1 -> Out/1

== system autoTakeoff/Autonomous Controller /Auto Take-off/Enroute Indicator/one-way switch  ==
  In : Inport
  Memory4 : Memory  InheritSampleTime=on
  Switch8 : Switch  Criteria=u2 > Threshold
  Out : Outport
  wires:
  Memory4/1 -> Out/1, Switch8/3
  Switch8/1 -> Memory4/1
  In/1 -> Switch8/1, Switch8/2

== system autoTakeoff/Autonomous Controller /Auto Take-off/Velocity Indicator/one-way switch  ==
  In : Inport
  Memory4 : Memory  InheritSampleTime=on
  Switch8 : Switch  Criteria=u2 > Threshold
  Out : Outport
  wires:
  Memory4/1 -> Out/1, Switch8/3
  Switch8/1 -> Memory4/1
  In/1 -> Switch8/1, Switch8/2

== matlab function autoTakeoff/Send to XPlane10/'DATA0' ==
  data: y output
function y = fcn()
%#codegen
%y=uint8(zeros(1,77));
y = uint8('DATA0');

== matlab function autoTakeoff/Get data from XPlane/MATLAB Function ==
  data: u input; Data output single size=[30 8]; msgLen input
function Data  = fcn(u,msgLen)
%#codegen
%coder.extrinsic('clear')
dataLen=msgLen-5;
Npackets=dataLen/36;

% initialize data matrix
% rows: packets of data; columns: data values, first column is the data
% index
maxNPackets=30;
Nvalues=8;% number of values in each packet
Data=single(zeros(maxNPackets,Nvalues));

Bytecounter=6; % start after the 5th byte

for i=1:msgLen
    
    if char(u(i))=='D' && char(u(i+1))=='A'
        %loop over each packet
        for j=1:Npackets
                indx=typecast(u(Bytecounter:Bytecounter+3),'uint32');% packet index
                %Data(indx,1)=single(indx); % packet index
                Bytecounter=Bytecounter+4; % go to the next 4 bytes
                Data(indx,1)=typecast(u(Bytecounter:Bytecounter+3),'single'); % 1st value
                Bytecounter=Bytecounter+4; % go to the next 4 bytes
                Data(indx,2)=typecast(u(Bytecounter:Bytecounter+3),'single'); % 2nd value
                Bytecounter=Bytecounter+4; % go to the next 4 bytes
                Data(indx,3)=typecast(u(Bytecounter:Bytecounter+3),'single'); % 3rd value
                Bytecounter=Bytecounter+4; % go to the next 4 bytes
                Data(indx,4)=typecast(u(Bytecounter:Bytecounter+3),'single'); % 4th value
                Bytecounter=Bytecounter+4; % go to the next 4 bytes
                Data(indx,5)=typecast(u(Bytecounter:Bytecounter+3),'single'); % 5th value
                Bytecounter=Bytecounter+4; % go to the next 4 bytes
                Data(indx,6)=typecast(u(Bytecounter:Bytecounter+3),'single'); % 6th value
                Bytecounter=Bytecounter+4; % go to the next 4 bytes
                Data(indx,7)=typecast(u(Bytecounter:Bytecounter+3),'single'); % 7th value
                Bytecounter=Bytecounter+4; % go to the next 4 bytes
                Data(indx,8)=typecast(u(Bytecounter:Bytecounter+3),'single'); % 8th value
                Bytecounter=Bytecounter+4;% go to the next packet index 
        end
        break
    end
end
%clear Data

== matlab function autoTakeoff/MATLAB Function1 ==
  data: AirportCoordinates output
function AirportCoordinates = getWP()
AirportCoordinates = [21.219041824340820 105.8135528564453 50; 21.225227355957030 105.7927398681641 50];
% AirportCoordinates = [21.219041824340820 105.8135528564453 50; 21.221620559692383 1.058050003051758e+02 50; 21.225227355957030 105.7927398681641 50];
% WPdataTable = [21.215 105.798 50; 21.219041824340820 105.8135528564453 50; 21.225227355957030 105.7927398681641 50];
% 21.220420837402344 1.058090286254883e+02;
% 21.221620559692383 1.058050003051758e+02;

== matlab function autoTakeoff/MATLAB Function2 ==
  data: WPdataTable output
function WPdataTable = getWP()
WPdataTable = [21.215 105.798 50; 21.219041824340820 105.8135528564453 50];
% WPdataTable = [21.215 105.798 50; 21.219041824340820 105.8135528564453 50; 21.225227355957030 105.7927398681641 50];
% 21.220420837402344 1.058090286254883e+02;
% 21.221620559692383 1.058050003051758e+02;
